simulink model "Response_Animations"  (R2025b)
settings: Solver=VariableStepAuto  StartTime=0.0  StopTime=15  RelTol=1e-3
libraries: aerolibanim x1
settings Model: Creator=maxma  LastModifiedBy=maxma

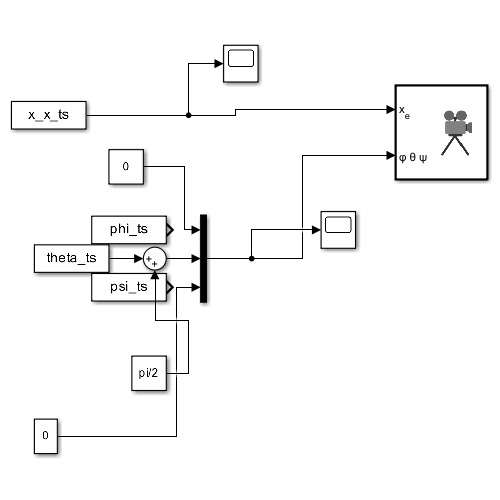
[thumbnail: Simulink's stored preview of the top-level diagram]
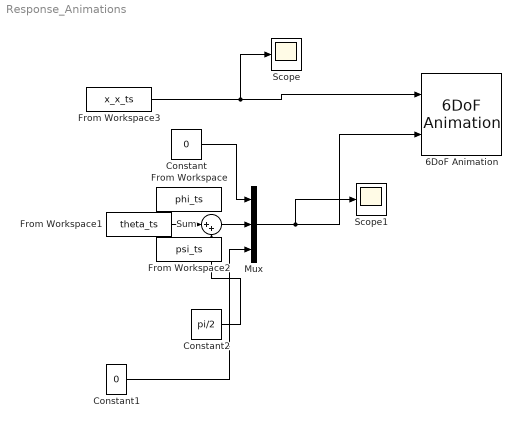
== system Response_Animations ==
  6DoF Animation : aerolibanim/6DoF Animation  u1=[-10 10 -10 10 -10 10]  u2=0.1  u3=1  u4=[4000 0 -5000]  u5=Fixed position  u6=[10 -10 0]  u7=5  u8=on
  Constant : Constant  Value=0
  Constant1 : Constant  Value=0
  Constant2 : Constant  Value=pi/2
  From Workspace : FromWorkspace  VariableName=phi_ts
  From Workspace1 : FromWorkspace  VariableName=theta_ts
  From Workspace2 : FromWorkspace  VariableName=psi_ts
  From Workspace3 : FromWorkspace  VariableName=x_x_ts
  Mux : Mux  Inputs=3
  Scope : Scope
      settings: ActiveDisplayYMinimum=-0.67490977103005867  ActiveDisplayYMaximum=1.5825903740535947
  Scope1 : Scope
      settings: ActiveDisplayYMinimum=-0.19634954084936201  ActiveDisplayYMaximum=1.7671458676442586
  Sum : Sum  Inputs=|++
  wires:
  Mux/1 -> Scope1/1, 6DoF Animation/2
  From Workspace3/1 -> Scope/1, 6DoF Animation/1
  Constant/1 -> Mux/1
  Constant1/1 -> Mux/3
  From Workspace1/1 -> Sum/1
  Sum/1 -> Mux/2
  Constant2/1 -> Sum/2
